simulink library "ddm"  (R2021b)
settings: Solver=VariableStepAuto  StartTime=0.0  StopTime=10.0  RelTol=1e-3
undefined symbols (not defined in the file or in its folder): ENUM_ADASACCSTA_ERROR, ENUM_ADASACCSTA_OFF, ENUM_ADASACCSTA_STANDBY, ENUM_ADASISASTA_OFF, ENUM_ALLOWMOV_ALLOWREADY, ENUM_APS, ENUM_BRKSTA_ERROR, ENUM_BRKSTA_OFF, ENUM_BRKSTA_ON, ENUM_BRKSW_INVALID, ENUM_BRKSW_OFF, ENUM_BRKSW_ON, ENUM_CHGPREACTERRSTA_OBCPRE, ENUM_DCDCFAULTSTA_ANYFAULTLV1, ENUM_DCDCFAULTSTA_ANYFAULTLV2, ENUM_DRIVETRAIN_AWD, ENUM_DRIVETRAIN_FWD, ENUM_DRIVETRAIN_RWD, ENUM_DRSEATSTA_INVALID, ENUM_EDUDRTSTA_NORMAL, ENUM_EPBSTA_APPLIED, ENUM_EPBSTA_RELEASED, ENUM_HVBATTREADYPRE_READY, ENUM_MCUWARN_LV0, ENUM_MCUWARN_LV1, ENUM_MCUWARN_LV2, ENUM_MCUWARN_LV3, ENUM_MCUWARN_NOERROR, ENUM_OBCFAULTSTA_ANYFAULT, ENUM_PAS_R2F2, ENUM_PDFAULT_BATTPDFAIL, ENUM_PDFAULT_DCDCDISABLE, ENUM_PDFAULT_MCUDISABLE, ENUM_PDFAULT_MCUDISCHRG, ENUM_POWERSTA_OFF, ENUM_POWERSTA_ON, ENUM_POWERSTA_READY, ENUM_POWERSTA_STANDBY, ENUM_PRESSINDI_LOW, ENUM_PUFAULT_BATTUPFAIL, ENUM_PUFAULT_DCDCENABLEFAIL, ENUM_PUFAULT_PRECHRGCHKFAIL, ENUM_PUFAULT_SAFETYCHKFAIL, ENUM_PUSTATE_COMPLETED, ENUM_PWRSTASW_OFF, ENUM_PWRSTASW_OFFA, ENUM_PWRSTASW_OFFCHVCHRG, ENUM_PWRSTASW_OFFCLVCHRG, ENUM_PWRSTASW_ON, ENUM_PWRSTASW_ONHVCHRG, ENUM_PWRSTASW_READY, ENUM_PWRSTASW_STANDBY, ENUM_RANGESTA_12IN, ENUM_SHIFTCOMMAND_D, ENUM_SHIFTCOMMAND_N, ENUM_SHIFTCOMMAND_P, ENUM_SHIFTCOMMAND_R, ENUM_VEHMALFUNLV_2ND, ENUM_VEHMALFUNLV_3RD, ENUM_VEHMALFUNLV_4TH ... (+835)
libraries: hcu_lib x750, $bdroot x12, simulink x5
(part 19 of 28)

== system ddm/DDM/DDM/PMM/LV/LV power supply voltage too high ==
  note: Diagnostics and Fault Handling
  note: Release Condition After Decision
  note: Test Pass Criteria
  note: Fail Safe After Decision
  note: Test Detection Criteria
  note: Fail Safe During Detection
  note: Release Condition During Detection
  task_time_s : Inport
  VPMM_PowerSta_enum : Inport  Port=2
  VPMM_PwrStaSW_enum : Inport  Port=3
  VINP_LVBattDet12V_V : Inport  Port=4
  VINP_CANMsgValidBMS2_flg : Inport  Port=5
  DTC_clear_request : Inport  Port=6
  Constant1 : Constant  Value=TRUE
  Constant10 : Constant  Value=ENUM_POWERSTA_OFF
  Constant11 : Constant  Value=KDDM_LVSupHiPassSW_flg
  Constant12 : Constant  Value=ENUM_PWRSTASW_READY
  Constant13 : Constant  Value=ENUM_PWRSTASW_ON
  Constant14 : Constant  Value=ENUM_PWRSTASW_OFFCLVCHRG
  Constant15 : Constant  Value=KDDM_LVSupHiCFSSW_flg
  Constant16 : Constant  Value=TRUE
  Constant17 : Constant  Value=ENUM_PWRSTASW_OFFCHVCHRG
  Constant18 : Constant  Value=KDDM_LVSupHiPassTO_s
  Constant19 : Constant  Value=KDDM_LVSupHiPassTO_s
  Constant2 : Constant  Value=ENUM_PWRSTASW_ON
  Constant20 : Constant  Value=KDDM_LVSupHiDFSSW_flg
  Constant{4,21,25,27} (4 alike) : Constant  Value=FALSE
  Constant22 : Constant  Value=ENUM_PWRSTASW_OFFCLVCHRG
  Constant23 : Constant  Value=ENUM_PWRSTASW_ONHVCHRG
  Constant24 : Constant  Value=TRUE
  Constant26 : Constant  Value=ENUM_PWRSTASW_OFFA
  Constant3 : Constant  Value=ENUM_PWRSTASW_ONHVCHRG
  Constant40 : Constant  Value=KDDM_LVSupHiDTC_cnt
  Constant41 : Constant  Value=KDDM_LVSupHiDetTO_s
  Constant46 : Constant  Value=KDDM_LVSupHiDetSW_flg
  Constant48 : Constant  Value=KDDM_LVSupHiDTC_cnt
  Constant5 : Constant  Value=ENUM_PWRSTASW_READY
  Constant6 : Constant  Value=KDDM_LVSupHiThd_mv
  Constant7 : Constant  Value=ENUM_PWRSTASW_OFFCHVCHRG
  Constant8 : Constant  Value=ENUM_PWRSTASW_OFFA
  Constant9 : Constant  Value=KDDM_LVSupHiThd_mv
  DTC_Couter : hcu_lib/Basic_Blocks/DTC_Couter
  DTC_Info : hcu_lib/Basic_Blocks/DTC_Info
  Data Type Conversion1 : DataTypeConversion  OutDataTypeStr=uint8
  Equal{,1..2,4,6,8..15} (13 alike) : RelationalOperator  Operator===  OutDataTypeStr=boolean  RndMeth=Simplest
  Equal3 : RelationalOperator  OutDataTypeStr=boolean  RndMeth=Simplest
  Equal5 : RelationalOperator  OutDataTypeStr=boolean  RndMeth=Simplest
  Equal7 : RelationalOperator  OutDataTypeStr=boolean  RndMeth=Simplest
  Gain1 : Gain  Gain=KXX2XX
  Gain2 : Gain  Gain=KXX2XX
  Goto6 : Goto  Commented=on  GotoTag=VDDM_EDriveSysErrVCUErr_flg
  Logical Operator{1..2,12,15,18} (5 alike) : Logic  AllPortsSameDT=off  OutDataTypeStr=boolean
  Logical Operator19 : Logic  Inputs=3  AllPortsSameDT=off  OutDataTypeStr=boolean
  Logical Operator3 : Logic  Operator=OR  Inputs=3  AllPortsSameDT=off  OutDataTypeStr=boolean
  Logical Operator4 : Logic  Operator=NOT  AllPortsSameDT=off  OutDataTypeStr=boolean
  Logical Operator5 : Logic  Operator=OR  AllPortsSameDT=off  OutDataTypeStr=boolean
  Logical Operator6 : Logic  Operator=NOT  AllPortsSameDT=off  OutDataTypeStr=boolean
  Logical Operator7 : Logic  Operator=OR  AllPortsSameDT=off  OutDataTypeStr=boolean
  Logical Operator8 : Logic  Operator=OR  AllPortsSameDT=off  OutDataTypeStr=boolean
  OR : Logic  Operator=OR  Inputs=6  AllPortsSameDT=off  OutDataTypeStr=boolean
  OR1 : Logic  Operator=OR  Inputs=6  AllPortsSameDT=off  OutDataTypeStr=boolean
  Relay : Relay  OnSwitchValue=ONE_INT  OffSwitchValue=ZERO_INT
  SR_Latch1 : Subsystem  mask(SR_Latch){}
      mask help: SR latch function.
  SR_Latch3 : hcu_lib/Basic_Blocks/SR_Latch
  SR_Latch4 : hcu_lib/Basic_Blocks/SR_Latch
  Switch{,2..4,6} (5 alike) : Switch  Criteria=u2 ~= 0
  Test Detection Criteria : hcu_lib/Basic_Blocks/Test Detection Criteria
  Timer1 : hcu_lib/Basic_Blocks/Timer
  VDDM_LVSupHiDTC_raw32 : Outport
  wires:
  DTC_Couter/2 -> Data Type Conversion1/1
  [DTC_clear_request] -> Logical Operator7/2
  Logical Operator5/1 -> SR_Latch4/2
  Logical Operator18/1 -> [VDDM_LVSupHiCFS_flg]  "VDDM_LVSupHiCFS_flg"
  Logical Operator7/1 -> SR_Latch3/2
  [DTC_clear_request] -> Logical Operator4/1
  [DTC_clear_request] -> Logical Operator5/2
  Logical Operator3/1 -> Logical Operator15/1
  Constant48/1 -> DTC_Couter/3
  [DTC_clear_request] -> Logical Operator3/3
  Logical Operator4/1 -> Logical Operator19/3
  [VDDM_LVSupHiCFS_flg] -> Logical Operator7/1
  [VDDM_LVSupHiDTC_cnt] -> Relay/1
  Constant15/1 -> Logical Operator18/2
  DTC_Couter/1 -> SR_Latch4/1
  Logical Operator12/1 -> [VDDM_LVSupHiDFS_flg]  "VDDM_LVSupHiDFS_flg"
  Logical Operator15/1 -> DTC_Couter/2
  [VDDM_LVSupHiCFSRls_flg] -> Logical Operator3/2
  Data Type Conversion1/1 -> [VDDM_LVSupHiDTC_cnt]  "VDDM_LVSupHiDTC_cnt"
  Constant46/1 -> Logical Operator19/2
  Relay/1 -> SR_Latch3/1
  SR_Latch4/1 -> Logical Operator18/1
  [VDDM_LVSupHiPass_flg] -> Logical Operator3/1
  Logical Operator19/1 -> DTC_Couter/1
  [VDDM_LVSupHiDet_flg] -> Logical Operator19/1
  Constant20/1 -> Logical Operator12/1
  [VDDM_LVSupHiCFSRls_flg] -> Logical Operator5/1
  SR_Latch3/1 -> Logical Operator12/2
  Constant11/1 -> Logical Operator15/2
  [VDDM_xxx_flg] -> SR_Latch1/2(reset)
  Constant27/1 -> Switch6/1
  Switch3/1 -> Switch6/3, [VDDM_xxx_flg]
  Switch6/1 -> Test Detection Criteria/1
  [DTC_clear_request] -> Switch6/2
  [DTC_clear_request] -> DTC_Info/4
  Constant7/1 -> Equal10/1
  Equal14/1 -> OR1/4
  [VPMM_PwrStaSW_enum] -> Equal2/1, Equal6/2
  Constant13/1 -> Equal6/1
  Logical Operator1/1 -> Switch4/2
  Equal15/1 -> OR1/3
  Constant5/1 -> Equal15/1
  [VPMM_PwrStaSW_enum] -> Equal14/1, Equal15/2
  OR1/1 -> Logical Operator1/1
  Equal6/1 -> OR1/1
  [VINP_CANMsgValidBMS2_flg] -> Logical Operator1/2
  Equal2/1 -> OR1/2
  Constant26/1 -> Equal14/2
  Constant23/1 -> Equal2/2
  Equal11/1 -> OR1/6
  [VPMM_PwrStaSW_enum] -> Equal11/1, Equal10/2
  Constant14/1 -> Equal11/2
  Equal10/1 -> OR1/5
  Constant17/1 -> Equal12/1
  Equal8/1 -> OR/4
  [VPMM_PwrStaSW_enum] -> Equal/1, Equal1/2
  Constant2/1 -> Equal1/1
  Logical Operator2/1 -> Switch3/2
  Equal9/1 -> OR/3
  Constant12/1 -> Equal9/1
  [VPMM_PwrStaSW_enum] -> Equal8/1, Equal9/2
  OR/1 -> Logical Operator2/1
  Equal1/1 -> OR/1
  [VINP_CANMsgValidBMS2_flg] -> Logical Operator2/2
  Equal/1 -> OR/2
  Constant8/1 -> Equal8/2
  Constant3/1 -> Equal/2
  Equal13/1 -> OR/6
  [VPMM_PwrStaSW_enum] -> Equal13/1, Equal12/2
  Constant22/1 -> Equal13/2
  Equal12/1 -> OR/5
  Constant41/1 -> Test Detection Criteria/4
  [VDDM_LVSupHiDet_flg] -> DTC_Info/1
  [VDDM_LVSupHiCFS_flg] -> DTC_Info/3
  [VDDM_LVSupHiPass_flg] -> DTC_Info/2
  DTC_Info/1 -> VDDM_LVSupHiDTC_raw32/1  "VDDM_LVSupHiDTC_raw32"
  VPMM_PwrStaSW_enum/1 -> [VPMM_PwrStaSW_enum]
  VPMM_PowerSta_enum/1 -> [VPMM_PowerSta_enum]
  [task_time_s] -> Timer1/3
  Constant6/1 -> Equal5/2
  Constant19/1 -> Equal3/2
  Logical Operator6/1 -> Timer1/1
  [VPMM_PowerSta_enum] -> Equal4/1
  Equal5/1 -> Switch3/1
  Constant25/1 -> Switch2/3
  Constant16/1 -> Switch4/3
  [DTC_clear_request] -> Logical Operator8/2
  Equal7/1 -> Switch4/1
  Gain1/1 -> Equal5/1
  Switch2/1 -> [VDDM_LVSupHiCFSRls_flg]  "VDDM_LVSupHiCFSRls_flg"
  [VINP_LVBattDet12V_V] -> Gain1/1
  Constant18/1 -> Timer1/4
  [VINP_LVBattDet12V_V] -> Gain2/1
  Gain2/1 -> Equal7/1
  Constant9/1 -> Equal7/2
  Constant40/1 -> Test Detection Criteria/3
  Constant1/1 -> Switch/1
  Switch4/1 -> Timer1/2, Logical Operator6/1
  Logical Operator8/1 -> Switch2/2
  Constant24/1 -> Switch2/1
  Constant10/1 -> Equal4/2
  Constant21/1 -> Switch/3
  [VDDM_LVSupHiCFS_flg] -> Switch/2
  Equal4/1 -> Logical Operator8/1
  Switch/1 -> Goto6/1
  Timer1/1 -> Equal3/1
  [task_time_s] -> Test Detection Criteria/2
  Test Detection Criteria/1 -> [VDDM_LVSupHiDet_flg]  "VDDM_LVSupHiDet_flg"
  Constant4/1 -> Switch3/3
  SR_Latch1/1(latched) -> [VDDM_LVSupHiPass_flg]  "VDDM_LVSupHiPass_flg"
  Equal3/1 -> SR_Latch1/1(set)
  VINP_CANMsgValidBMS2_flg/1 -> [VINP_CANMsgValidBMS2_flg]
  DTC_clear_request/1 -> [DTC_clear_request]
  VINP_LVBattDet12V_V/1 -> [VINP_LVBattDet12V_V]
  task_time_s/1 -> [task_time_s]

== system ddm/DDM/DDM/PMM/LV/LV power supply voltage too low ==
  note: Diagnostics and Fault Handling
  note: Release Condition After Decision
  note: Release Condition During Detection
  note: Fail Safe During Detection
  note: Fail Safe After Decision
  note: Test Pass Criteria
  note: Test Detection Criteria
  task_time_s : Inport
  VPMM_PowerSta_enum : Inport  Port=2
  VPMM_PwrStaSW_enum : Inport  Port=3
  VINP_LVBattDet12V_V : Inport  Port=4
  VINP_CANMsgValidBMS2_flg : Inport  Port=5
  DTC_clear_request : Inport  Port=6
  Constant1 : Constant  Value=TRUE
  Constant10 : Constant  Value=ENUM_POWERSTA_OFF
  Constant11 : Constant  Value=KDDM_LVSupLoPassSW_flg
  Constant12 : Constant  Value=ENUM_PWRSTASW_READY
  Constant13 : Constant  Value=ENUM_PWRSTASW_ON
  Constant14 : Constant  Value=ENUM_PWRSTASW_OFFCLVCHRG
  Constant15 : Constant  Value=KDDM_LVSupLoCFSSW_flg
  Constant16 : Constant  Value=TRUE
  Constant17 : Constant  Value=ENUM_PWRSTASW_OFFCHVCHRG
  Constant18 : Constant  Value=KDDM_LVSupLoPassTO_s
  Constant19 : Constant  Value=KDDM_LVSupLoPassTO_s
  Constant2 : Constant  Value=ENUM_PWRSTASW_ON
  Constant20 : Constant  Value=KDDM_LVSupLoDFSSW_flg
  Constant{4,21,25,27} (4 alike) : Constant  Value=FALSE
  Constant22 : Constant  Value=ENUM_PWRSTASW_OFFCLVCHRG
  Constant23 : Constant  Value=ENUM_PWRSTASW_ONHVCHRG
  Constant24 : Constant  Value=TRUE
  Constant26 : Constant  Value=ENUM_PWRSTASW_OFFA
  Constant3 : Constant  Value=ENUM_PWRSTASW_ONHVCHRG
  Constant40 : Constant  Value=KDDM_LVSupLoDTC_cnt
  Constant41 : Constant  Value=KDDM_LVSupLoDetTO_s
  Constant46 : Constant  Value=KDDM_LVSupLoDetSW_flg
  Constant48 : Constant  Value=KDDM_LVSupLoDTC_cnt
  Constant5 : Constant  Value=ENUM_PWRSTASW_READY
  Constant6 : Constant  Value=KDDM_LVSupLoThd_mv
  Constant7 : Constant  Value=ENUM_PWRSTASW_OFFCHVCHRG
  Constant8 : Constant  Value=ENUM_PWRSTASW_OFFA
  Constant9 : Constant  Value=KDDM_LVSupLoThd_mv
  DTC_Couter : hcu_lib/Basic_Blocks/DTC_Couter
  DTC_Info : hcu_lib/Basic_Blocks/DTC_Info
  Data Type Conversion1 : DataTypeConversion  OutDataTypeStr=uint8
  Equal{,1..2,4,6,8..15} (13 alike) : RelationalOperator  Operator===  OutDataTypeStr=boolean  RndMeth=Simplest
  Equal3 : RelationalOperator  OutDataTypeStr=boolean  RndMeth=Simplest
  Equal5 : RelationalOperator  Operator=<=  OutDataTypeStr=boolean  RndMeth=Simplest
  Equal7 : RelationalOperator  Operator=<=  OutDataTypeStr=boolean  RndMeth=Simplest
  Gain1 : Gain  Gain=1000
  Gain2 : Gain  Gain=1000
  Goto6 : Goto  Commented=on  GotoTag=VDDM_EDriveSysErrVCUErr_flg
  Logical Operator{1..2,12,15,18} (5 alike) : Logic  AllPortsSameDT=off  OutDataTypeStr=boolean
  Logical Operator19 : Logic  Inputs=3  AllPortsSameDT=off  OutDataTypeStr=boolean
  Logical Operator3 : Logic  Operator=OR  Inputs=3  AllPortsSameDT=off  OutDataTypeStr=boolean
  Logical Operator4 : Logic  Operator=NOT  AllPortsSameDT=off  OutDataTypeStr=boolean
  Logical Operator5 : Logic  Operator=OR  AllPortsSameDT=off  OutDataTypeStr=boolean
  Logical Operator6 : Logic  Operator=NOT  AllPortsSameDT=off  OutDataTypeStr=boolean
  Logical Operator7 : Logic  Operator=OR  AllPortsSameDT=off  OutDataTypeStr=boolean
  Logical Operator8 : Logic  Operator=OR  AllPortsSameDT=off  OutDataTypeStr=boolean
  OR : Logic  Operator=OR  Inputs=6  AllPortsSameDT=off  OutDataTypeStr=boolean
  OR1 : Logic  Operator=OR  Inputs=6  AllPortsSameDT=off  OutDataTypeStr=boolean
  Relay : Relay  OnSwitchValue=ONE_INT  OffSwitchValue=ZERO_INT
  SR_Latch1 : Subsystem  mask(SR_Latch){}
      mask help: SR latch function.
  SR_Latch3 : hcu_lib/Basic_Blocks/SR_Latch
  SR_Latch4 : hcu_lib/Basic_Blocks/SR_Latch
  Switch{,2..4,6} (5 alike) : Switch  Criteria=u2 ~= 0
  Test Detection Criteria : hcu_lib/Basic_Blocks/Test Detection Criteria
  Timer1 : hcu_lib/Basic_Blocks/Timer
  VDDM_LVSupLoDTC_raw32 : Outport
  wires:
  Constant46/1 -> Logical Operator19/2
  Logical Operator12/1 -> [VDDM_LVSupLoDFS_flg]  "VDDM_LVSupLoDFS_flg"
  Logical Operator5/1 -> SR_Latch4/2
  [VDDM_LVSupLoPass_flg] -> Logical Operator3/1
  Constant11/1 -> Logical Operator15/2
  Data Type Conversion1/1 -> [VDDM_LVSupLoDTC_cnt]  "VDDM_LVSupLoDTC_cnt"
  [DTC_clear_request] -> Logical Operator4/1
  SR_Latch3/1 -> Logical Operator12/2
  Logical Operator4/1 -> Logical Operator19/3
  Constant20/1 -> Logical Operator12/1
  Logical Operator19/1 -> DTC_Couter/1
  Logical Operator18/1 -> [VDDM_LVSupLoCFS_flg]  "VDDM_LVSupLoCFS_flg"
  [DTC_clear_request] -> Logical Operator5/2
  DTC_Couter/2 -> Data Type Conversion1/1
  Logical Operator3/1 -> Logical Operator15/1
  Constant48/1 -> DTC_Couter/3
  [VDDM_LVSupLoDet_flg] -> Logical Operator19/1
  [VDDM_LVSupLoDTC_cnt] -> Relay/1
  [DTC_clear_request] -> Logical Operator3/3
  Logical Operator7/1 -> SR_Latch3/2
  [VDDM_LVSupLoCFS_flg] -> Logical Operator7/1
  Logical Operator15/1 -> DTC_Couter/2
  Relay/1 -> SR_Latch3/1
  DTC_Couter/1 -> SR_Latch4/1
  SR_Latch4/1 -> Logical Operator18/1
  Constant15/1 -> Logical Operator18/2
  [DTC_clear_request] -> Logical Operator7/2
  [VDDM_LVSupLoCFSRls_flg] -> Logical Operator3/2
  [VDDM_LVSupLoCFSRls_flg] -> Logical Operator5/1
  [VDDM_xxx_flg] -> SR_Latch1/2(reset)
  Constant27/1 -> Switch6/1
  Switch3/1 -> Switch6/3, [VDDM_xxx_flg]
  Switch6/1 -> Test Detection Criteria/1
  [DTC_clear_request] -> Switch6/2
  [DTC_clear_request] -> DTC_Info/4
  Constant7/1 -> Equal10/1
  Equal14/1 -> OR1/4
  [VPMM_PwrStaSW_enum] -> Equal2/1, Equal6/2
  Constant13/1 -> Equal6/1
  Logical Operator1/1 -> Switch4/2
  Equal15/1 -> OR1/3
  Constant5/1 -> Equal15/1
  [VPMM_PwrStaSW_enum] -> Equal14/1, Equal15/2
  OR1/1 -> Logical Operator1/1
  Equal6/1 -> OR1/1
  [VINP_CANMsgValidBMS2_flg] -> Logical Operator1/2
  Equal2/1 -> OR1/2
  Constant26/1 -> Equal14/2
  Constant23/1 -> Equal2/2
  Equal11/1 -> OR1/6
  [VPMM_PwrStaSW_enum] -> Equal11/1, Equal10/2
  Constant14/1 -> Equal11/2
  Equal10/1 -> OR1/5
  Equal13/1 -> OR/6
  Equal12/1 -> OR/5
  Constant22/1 -> Equal13/2
  Constant17/1 -> Equal12/1
  [VPMM_PwrStaSW_enum] -> Equal13/1, Equal12/2
  Constant41/1 -> Test Detection Criteria/4
  [VDDM_LVSupLoDet_flg] -> DTC_Info/1
  [VDDM_LVSupLoCFS_flg] -> DTC_Info/3
  [VDDM_LVSupLoPass_flg] -> DTC_Info/2
  DTC_Info/1 -> VDDM_LVSupLoDTC_raw32/1  "VDDM_LVSupLoDTC_raw32"
  [VPMM_PowerSta_enum] -> Equal4/1
  [task_time_s] -> Timer1/3
  Equal8/1 -> OR/4
  Equal9/1 -> OR/3
  Constant12/1 -> Equal9/1
  [VPMM_PwrStaSW_enum] -> Equal8/1, Equal9/2
  Constant8/1 -> Equal8/2
  Constant9/1 -> Equal7/2
  [VINP_LVBattDet12V_V] -> Gain2/1
  Gain2/1 -> Equal7/1
  Equal7/1 -> Switch4/1
  Gain1/1 -> Equal5/1
  Constant6/1 -> Equal5/2
  Equal5/1 -> Switch3/1
  [VINP_LVBattDet12V_V] -> Gain1/1
  Constant2/1 -> Equal1/1
  Equal1/1 -> OR/1
  OR/1 -> Logical Operator2/1
  Equal/1 -> OR/2
  [VINP_CANMsgValidBMS2_flg] -> Logical Operator2/2
  VINP_CANMsgValidBMS2_flg/1 -> [VINP_CANMsgValidBMS2_flg]
  DTC_clear_request/1 -> [DTC_clear_request]
  Equal4/1 -> Logical Operator8/1
  Constant10/1 -> Equal4/2
  Constant24/1 -> Switch2/1
  [DTC_clear_request] -> Logical Operator8/2
  Switch2/1 -> [VDDM_LVSupLoCFSRls_flg]  "VDDM_LVSupLoCFSRls_flg"
  Constant25/1 -> Switch2/3
  Logical Operator8/1 -> Switch2/2
  Constant21/1 -> Switch/3
  Constant1/1 -> Switch/1
  Switch/1 -> Goto6/1
  [VDDM_LVSupLoCFS_flg] -> Switch/2
  Constant16/1 -> Switch4/3
  Constant18/1 -> Timer1/4
  Timer1/1 -> Equal3/1
  Switch4/1 -> Timer1/2, Logical Operator6/1
  Constant19/1 -> Equal3/2
  Logical Operator6/1 -> Timer1/1
  Equal3/1 -> SR_Latch1/1(set)
  SR_Latch1/1(latched) -> [VDDM_LVSupLoPass_flg]  "VDDM_LVSupLoPass_flg"
  [VPMM_PwrStaSW_enum] -> Equal/1, Equal1/2
  Constant4/1 -> Switch3/3
  Constant3/1 -> Equal/2
  Constant40/1 -> Test Detection Criteria/3
  Test Detection Criteria/1 -> [VDDM_LVSupLoDet_flg]  "VDDM_LVSupLoDet_flg"
  [task_time_s] -> Test Detection Criteria/2
  Logical Operator2/1 -> Switch3/2
  VPMM_PowerSta_enum/1 -> [VPMM_PowerSta_enum]
  VPMM_PwrStaSW_enum/1 -> [VPMM_PwrStaSW_enum]
  VINP_LVBattDet12V_V/1 -> [VINP_LVBattDet12V_V]
  task_time_s/1 -> [task_time_s]

== system ddm/DDM/DDM/PMM/SW failure/Driver seat switch failure ==
  note: Diagnostics and Fault Handling
  note: Release Condition During Detection
  note: Release Condition After Decision
  note: Fail Safe After Decision
  note: Fail Safe During Detection
  note: Test Detection Criteria
  note: Test Pass Criteria
  task_time_s : Inport
  VPMM_PowerSta_enum : Inport  Port=2
  VPMM_PwrStaSW_enum : Inport  Port=3
  VINP_DrStSW : Inport  Port=4
  DTC_clear_request : Inport  Port=5
  Constant15 : Constant  Value=KDDM_DrStSWDetTO_s
  Constant16 : Constant  Value=KDDM_DrStSWDTC_cnt
  Constant17 : Constant  Value=KDDM_DrStSWPassTO_s
  Constant18 : Constant  Value=FALSE
  Constant19 : Constant  Value=ENUM_PWRSTASW_OFF
  Constant20 : Constant  Value=KDDM_DrStSWPassTO_s
  Constant21 : Constant  Value=ZERO_INT
  Constant22 : Constant  Value=ENUM_PWRSTASW_OFF
  Constant23 : Constant  Value=TRUE
  Constant24 : Constant  Value=KDDM_DrStSWPassTO_s
  Constant26 : Constant  Value=ONE_INT
  Constant27 : Constant  Value=KDDM_DrStSW_s
  Constant42 : Constant  Value=ENUM_DRSEATSTA_INVALID
  Constant45 : Constant  Value=ENUM_POWERSTA_OFF
  Constant52 : Constant  Value=TRUE
  Constant53 : Constant  Value=FALSE
  Constant54 : Constant  Value=TRUE
  Constant55 : Constant  Value=FALSE
  Constant56 : Constant  Value=KDDM_DrStSWPassSW_flg
  Constant57 : Constant  Value=KDDM_DrStSWCFSSW_flg
  Constant58 : Constant  Value=KDDM_DrStSWDFSSW_flg
  Constant59 : Constant  Value=KDDM_DrStSWDetSW_flg
  Constant60 : Constant  Value=KDDM_DrStSWDTC_cnt
  Constant8 : Constant  Value=ZERO_FLOAT
  DTC_Couter1 : hcu_lib/Basic_Blocks/DTC_Couter
  DTC_Info : hcu_lib/Basic_Blocks/DTC_Info
  Data Type Conversion11 : DataTypeConversion
  Data Type Conversion12 : DataTypeConversion  OutDataTypeStr=boolean
  Data Type Conversion4 : DataTypeConversion  OutDataTypeStr=uint8
  Equal1 : RelationalOperator  Operator=~=  OutDataTypeStr=boolean  RndMeth=Simplest
  Equal2 : RelationalOperator  Operator=~=  OutDataTypeStr=boolean  RndMeth=Simplest
  Equal3 : RelationalOperator  Operator=~=  OutDataTypeStr=boolean  RndMeth=Simplest
  Equal5 : RelationalOperator  OutDataTypeStr=boolean  RndMeth=Simplest
  Equal8 : RelationalOperator  Operator===  OutDataTypeStr=boolean  RndMeth=Simplest
  Logical Operator{2,4..5,7} (4 alike) : Logic  Operator=NOT  AllPortsSameDT=off  OutDataTypeStr=boolean
  Logical Operator27 : Logic  Operator=OR  AllPortsSameDT=off  OutDataTypeStr=boolean
  Logical Operator{6,28..30} (4 alike) : Logic  AllPortsSameDT=off  OutDataTypeStr=boolean
  Logical Operator3 : Logic  Operator=OR  AllPortsSameDT=off  OutDataTypeStr=boolean
  Logical Operator31 : Logic  Inputs=3  AllPortsSameDT=off  OutDataTypeStr=boolean
  Logical Operator32 : Logic  Operator=OR  Inputs=3  AllPortsSameDT=off  OutDataTypeStr=boolean
  Logical Operator33 : Logic  Operator=OR  Inputs=3  AllPortsSameDT=off  OutDataTypeStr=boolean
  Relational Operator3 : RelationalOperator  Operator=>  OutDataTypeStr=boolean  RndMeth=Simplest
  Relational Operator4 : RelationalOperator  Operator=<=  OutDataTypeStr=boolean  RndMeth=Simplest
  Relay1 : Relay  OnSwitchValue=ONE_INT  OffSwitchValue=ZERO_INT
  SR_Latch1 : hcu_lib/Basic_Blocks/SR_Latch
  SR_Latch2 : hcu_lib/Basic_Blocks/SR_Latch
  SR_Latch3 : Subsystem  mask(SR_Latch){}
      mask help: SR latch function.
  SR_Latch5 : hcu_lib/Basic_Blocks/SR_Latch
  Subsystem : Subsystem
  Switch{5,10..11,14..16} (6 alike) : Switch  Criteria=u2 ~= 0
  Test Detection Criteria2 : hcu_lib/Basic_Blocks/Test Detection Criteria
  Timer : hcu_lib/Basic_Blocks/Test Detection Criteria/Timer
  Timer1 : hcu_lib/Basic_Blocks/Timer
  Unit Delay : UnitDelay  SampleTime=-1  HasFrameUpgradeWarning=on
  Unit Delay7 : UnitDelay  SampleTime=-1  HasFrameUpgradeWarning=on
  VDDM_DrStSWDTC_raw32 : Outport
  VDDM_DrSeatSta_enum : Outport  Port=2
  wires:
  [DTC_clear_request] -> Logical Operator32/3
  [DTC_clear_request] -> Logical Operator33/3
  [DTC_clear_request] -> Logical Operator3/2
  Constant57/1 -> Logical Operator30/2
  Logical Operator2/1 -> Logical Operator31/3
  Constant59/1 -> Logical Operator31/2
  Logical Operator3/1 -> SR_Latch5/2
  [DTC_clear_request] -> Logical Operator2/1
  Logical Operator28/1 -> [VDDM_DrStSWDFS_flg]  "VDDM_DrStSWDFS_flg"
  Logical Operator32/1 -> SR_Latch2/2
  DTC_Couter1/1 -> SR_Latch5/1
  [VDDM_DrStSWCFSRls_flg] -> Logical Operator33/2
  [VDDM_DrStSWDFSRls_flg] -> Logical Operator32/1
  SR_Latch5/1 -> Logical Operator30/1
  Logical Operator31/1 -> DTC_Couter1/1
  [VDDM_DrStSWDTC_cnt] -> Relay1/1
  Relay1/1 -> SR_Latch2/1
  SR_Latch2/1 -> Logical Operator28/2
  Constant60/1 -> DTC_Couter1/3
  [VDDM_DrStSWDet_flg] -> Logical Operator31/1
  [VDDM_DrStSWCFSRls_flg] -> Logical Operator3/1
  Logical Operator33/1 -> Logical Operator29/1
  Constant58/1 -> Logical Operator28/1
  Constant56/1 -> Logical Operator29/2
  [VDDM_DrStSWPass_flg] -> Logical Operator33/1
  Logical Operator29/1 -> DTC_Couter1/2
  DTC_Couter1/2 -> Data Type Conversion4/1
  Data Type Conversion4/1 -> [VDDM_DrStSWDTC_cnt]  "VDDM_DrStSWDTC_cnt"
  [VDDM_DrStSWCFS_flg] -> Logical Operator32/2
  Logical Operator30/1 -> [VDDM_DrStSWCFS_flg]  "VDDM_DrStSWCFS_flg"
  [DTC_clear_request] -> DTC_Info/4
  [VDDM_DrStSWDet_flg] -> DTC_Info/1
  [VDDM_DrStSWCFS_flg] -> DTC_Info/3
  [VDDM_DrStSWPass_flg] -> DTC_Info/2
  DTC_Info/1 -> VDDM_DrStSWDTC_raw32/1  "VDDM_DrStSWDTC_raw32"
  [VINP_DrStSWGPIO_flg] -> Switch11/3
  VPMM_PwrStaSW_enum/1 -> [VPMM_PwrStaSW_enum]
  VPMM_PowerSta_enum/1 -> [VPMM_PowerSta_enum]
  [VDDM_DrSeatSta_enum] -> VDDM_DrSeatSta_enum/1
  [VPMM_PowerSta_enum] -> Equal8/1
  Constant54/1 -> Switch15/1
  [DTC_clear_request] -> Logical Operator27/2
  Switch16/1 -> [VDDM_DrStSWDFSRls_flg]  "VDDM_DrStSWDFSRls_flg"
  Switch15/1 -> [VDDM_DrStSWCFSRls_flg]  "VDDM_DrStSWCFSRls_flg"
  Constant55/1 -> Switch15/3
  Constant45/1 -> Equal8/2
  Constant53/1 -> Switch16/3
  [VDDM_DrStSWPass_flg] -> Switch16/2
  Equal8/1 -> Logical Operator27/1
  Constant52/1 -> Switch16/1
  Logical Operator27/1 -> Switch15/2
  Switch11/1 -> [VDDM_DrSeatSta_enum]  "VDDM_DrSeatSta_enum"
  Constant42/1 -> Switch11/1
  [VDDM_DrStSWCFS_flg] -> Switch11/2
  task_time_s/1 -> [task_time_s]
  VINP_DrStSW/1 -> [VINP_DrStSWGPIO_flg]
  DTC_clear_request/1 -> [DTC_clear_request]
  SR_Latch1/1 -> Logical Operator5/1, Logical Operator4/1, Timer/1
  Constant17/1 -> Timer/4
  Timer/1 -> Relational Operator4/1, Unit Delay/1
  [VDDM_xxx_flg] -> SR_Latch3/2(reset)
  [DTC_clear_request] -> Switch5/2
  Switch5/1 -> Data Type Conversion12/1
  Constant18/1 -> Switch5/1
  Constant15/1 -> Data Type Conversion11/1
  Constant26/1 -> SR_Latch1/1
  Logical Operator5/1 -> Subsystem/Trigger
  Constant20/1 -> Equal5/2
  [DrStSWFault_flg] -> Switch10/1
  Switch14/1 -> [VDDM_xxx_flg], Switch5/3
  Test Detection Criteria2/1 -> [VDDM_DrStSWDet_flg]  "VDDM_DrStSWDet_flg"
  [VPMM_PwrStaSW_enum] -> Equal1/1
  Constant22/1 -> Equal1/2
  Constant21/1 -> Switch14/3
  Equal1/1 -> Switch14/2
  Data Type Conversion11/1 -> Test Detection Criteria2/4
  Equal2/1 -> [VDDM_DrStSWChange_flg]
  Logical Operator4/1 -> Timer/2
  Subsystem/1(Fault_flg) -> Logical Operator6/1
  [VDDM_DrStSWChange_flg] -> SR_Latch1/2
  Constant16/1 -> Test Detection Criteria2/3
  Relational Operator4/1 -> Logical Operator6/2
  [task_time_s] -> Test Detection Criteria2/2
  Logical Operator7/1 -> Timer1/1
  Equal3/1 -> Switch10/2
  Equal5/1 -> SR_Latch3/1(set)
  Switch10/1 -> Logical Operator7/1, Timer1/2
  SR_Latch3/1(latched) -> [VDDM_DrStSWPass_flg]  "VDDM_DrStSWPass_flg"
  Unit Delay/1 -> Subsystem/1(In1)
  Logical Operator6/1 -> [DrStSWFault_flg], Switch14/1
  Data Type Conversion12/1 -> Test Detection Criteria2/1
  Constant23/1 -> Switch10/3
  Constant19/1 -> Equal3/2
  Timer1/1 -> Equal5/1
  [task_time_s] -> Timer1/3
  [VPMM_PwrStaSW_enum] -> Equal3/1
  Constant8/1 -> Relational Operator3/2
  Unit Delay7/1 -> Equal2/1
  [VINP_DrStSWGPIO_flg] -> Relational Operator3/1
  Constant24/1 -> Timer1/4
  Relational Operator3/1 -> Equal2/2, Unit Delay7/1
  Constant27/1 -> Relational Operator4/2
  [task_time_s] -> Timer/3

== system ddm/DDM/DDM/PMM/SW failure/FL Door switch failure ==
  note: Diagnostics and Fault Handling
  note: Fail Safe During Detection
  note: Fail Safe After Decision
  note: Release Condition After Decision
  note: Release Condition During Detection
  note: Test Pass Criteria
  note: Test Detection Criteria
  task_time_s : Inport
  VPMM_PowerSta_enum : Inport  Port=2
  VPMM_PwrStaSW_enum : Inport  Port=3
  VINP_FLAJARSW : Inport  Port=4
  DTC_clear_request : Inport  Port=5
  Constant{10,18,53,55} (4 alike) : Constant  Value=FALSE
  Constant11 : Constant  Value=KDDM_FLDoorSWPassTO_s
  Constant15 : Constant  Value=KDDM_FLDoorSWPassTO_s
  Constant16 : Constant  Value=KDDM_FLDoorSWDetTO_s
  Constant17 : Constant  Value=KDDM_FLDoorSW_s
  Constant19 : Constant  Value=ENUM_PWRSTASW_OFF
  Constant21 : Constant  Value=ZERO_INT
  Constant22 : Constant  Value=ENUM_PWRSTASW_OFF
  Constant{23,42,52,54} (4 alike) : Constant  Value=TRUE
  Constant24 : Constant  Value=KDDM_FLDoorSWPassTO_s
  Constant25 : Constant  Value=KDDM_FLDoorSWDTC_cnt
  Constant26 : Constant  Value=ONE_INT
  Constant32 : Constant  Value=ZERO_FLOAT
  Constant45 : Constant  Value=ENUM_POWERSTA_OFF
  Constant56 : Constant  Value=KDDM_FLDoorSWPassSW_flg
  Constant57 : Constant  Value=KDDM_FLDoorSWCFSSW_flg
  Constant58 : Constant  Value=KDDM_FLDoorSWDFSSW_flg
  Constant59 : Constant  Value=KDDM_FLDoorSWDetSW_flg
  Constant60 : Constant  Value=KDDM_FLDoorSWDTC_cnt
  DTC_Couter1 : hcu_lib/Basic_Blocks/DTC_Couter
  DTC_Info : hcu_lib/Basic_Blocks/DTC_Info
  Data Type Conversion12 : DataTypeConversion  OutDataTypeStr=boolean
  Data Type Conversion14 : DataTypeConversion  OutDataTypeStr=boolean
  Data Type Conversion4 : DataTypeConversion  OutDataTypeStr=uint8
  Data Type Conversion7 : DataTypeConversion
  Equal1 : RelationalOperator  Operator=~=  OutDataTypeStr=boolean  RndMeth=Simplest
  Equal3 : RelationalOperator  Operator=~=  OutDataTypeStr=boolean  RndMeth=Simplest
  Equal4 : RelationalOperator  Operator=~=  OutDataTypeStr=boolean  RndMeth=Simplest
  Equal5 : RelationalOperator  OutDataTypeStr=boolean  RndMeth=Simplest
  Equal8 : RelationalOperator  Operator===  OutDataTypeStr=boolean  RndMeth=Simplest
  Logical Operator{2,4..5,7} (4 alike) : Logic  Operator=NOT  AllPortsSameDT=off  OutDataTypeStr=boolean
  Logical Operator27 : Logic  Operator=OR  AllPortsSameDT=off  OutDataTypeStr=boolean
  Logical Operator{6,28..30} (4 alike) : Logic  AllPortsSameDT=off  OutDataTypeStr=boolean
  Logical Operator3 : Logic  Operator=OR  AllPortsSameDT=off  OutDataTypeStr=boolean
  Logical Operator31 : Logic  Inputs=3  AllPortsSameDT=off  OutDataTypeStr=boolean
  Logical Operator32 : Logic  Operator=OR  Inputs=3  AllPortsSameDT=off  OutDataTypeStr=boolean
  Logical Operator33 : Logic  Operator=OR  Inputs=3  AllPortsSameDT=off  OutDataTypeStr=boolean
  Relational Operator4 : RelationalOperator  Operator=<=  OutDataTypeStr=boolean  RndMeth=Simplest
  Relational Operator5 : RelationalOperator  Operator=>  OutDataTypeStr=boolean  RndMeth=Simplest
  Relay1 : Relay  OnSwitchValue=ONE_INT  OffSwitchValue=ZERO_INT
  SR_Latch1 : hcu_lib/Basic_Blocks/SR_Latch
  SR_Latch2 : hcu_lib/Basic_Blocks/SR_Latch
  SR_Latch3 : $bdroot/DDM/DDM/PMM/SW failure/Driver seat switch failure/SR_Latch3
  SR_Latch5 : hcu_lib/Basic_Blocks/SR_Latch
  Subsystem : $bdroot/DDM/DDM/PMM/SW failure/Driver seat switch failure/Subsystem  SystemSampleTime=-1  VariantActivationTime=update diagram  Latency=0  AutoFrameSizeCalculation=off
      link override Constant15: Value=KDDM_FLDoorSW_s
  Switch{5,10..11,14..16} (6 alike) : Switch  Criteria=u2 ~= 0
  Test Detection Criteria2 : hcu_lib/Basic_Blocks/Test Detection Criteria
  Timer : hcu_lib/Basic_Blocks/Test Detection Criteria/Timer
  Timer1 : hcu_lib/Basic_Blocks/Timer
  Unit Delay : UnitDelay  SampleTime=-1  HasFrameUpgradeWarning=on
  Unit Delay9 : UnitDelay  SampleTime=-1  HasFrameUpgradeWarning=on
  VDDM_FLDoorSWDTC_raw32 : Outport
  VDDM_VCUFLDoorSta_flg : Outport  Port=2
  wires:
  [DTC_clear_request] -> Logical Operator3/2
  Logical Operator2/1 -> Logical Operator31/3
  [DTC_clear_request] -> Logical Operator32/3
  [DTC_clear_request] -> Logical Operator33/3
  Logical Operator29/1 -> DTC_Couter1/2
  [DTC_clear_request] -> Logical Operator2/1
  [VDDM_FLDoorSWDet_flg] -> Logical Operator31/1
  Logical Operator31/1 -> DTC_Couter1/1
  [VDDM_FLDoorSWDTC_cnt] -> Relay1/1
  Logical Operator33/1 -> Logical Operator29/1
  DTC_Couter1/1 -> SR_Latch5/1
  SR_Latch5/1 -> Logical Operator30/1
  SR_Latch2/1 -> Logical Operator28/2
  Data Type Conversion4/1 -> [VDDM_FLDoorSWDTC_cnt]  "VDDM_FLDoorSWDTC_cnt"
  DTC_Couter1/2 -> Data Type Conversion4/1
  Relay1/1 -> SR_Latch2/1
  [VDDM_FLDoorSWCFSRls_flg] -> Logical Operator3/1
  [VDDM_FLDoorSWCFS_flg] -> Logical Operator32/2
  Logical Operator28/1 -> [VDDM_FLDoorSWDFS_flg]  "VDDM_FLDoorSWDFS_flg"
  [VDDM_FLDoorSWPass_flg] -> Logical Operator33/1
  Constant60/1 -> DTC_Couter1/3
  [VDDM_FLDoorSWDFSRls_flg] -> Logical Operator32/1
  Constant56/1 -> Logical Operator29/2
  Constant58/1 -> Logical Operator28/1
  Logical Operator32/1 -> SR_Latch2/2
  Constant59/1 -> Logical Operator31/2
  [VDDM_FLDoorSWCFSRls_flg] -> Logical Operator33/2
  Logical Operator3/1 -> SR_Latch5/2
  Constant57/1 -> Logical Operator30/2
  Logical Operator30/1 -> [VDDM_FLDoorSWCFS_flg]  "VDDM_FLDoorSWCFS_flg"
  [DTC_clear_request] -> DTC_Info/4
  [VDDM_FLDoorSWDet_flg] -> DTC_Info/1
  [VDDM_FLDoorSWCFS_flg] -> DTC_Info/3
  [VDDM_FLDoorSWPass_flg] -> DTC_Info/2
  DTC_Info/1 -> VDDM_FLDoorSWDTC_raw32/1  "VDDM_FLDoorSWDTC_raw32"
  Constant10/1 -> Switch11/3
  VPMM_PowerSta_enum/1 -> [VPMM_PowerSta_enum]
  VPMM_PwrStaSW_enum/1 -> [VPMM_PwrStaSW_enum]
  DTC_clear_request/1 -> [DTC_clear_request]
  VINP_FLAJARSW/1 -> [VINP_FL_AJAR_SW]
  task_time_s/1 -> [task_time_s]
  [VDDM_FLDoorSWCFS_flg] -> Switch11/2
  Constant42/1 -> Switch11/1
  Switch11/1 -> [VDDM_VCUFLDoorSta_flg]  "VDDM_VCUFLDoorSta_flg"
  Logical Operator27/1 -> Switch15/2
  Constant52/1 -> Switch16/1
  Equal8/1 -> Logical Operator27/1
  [VDDM_FLDoorSWPass_flg] -> Switch16/2
  Constant53/1 -> Switch16/3
  Constant45/1 -> Equal8/2
  Constant55/1 -> Switch15/3
  Switch15/1 -> [VDDM_FLDoorSWCFSRls_flg]  "VDDM_FLDoorSWCFSRls_flg"
  Switch16/1 -> [VDDM_FLDoorSWDFSRls_flg]  "VDDM_FLDoorSWDFSRls_flg"
  [DTC_clear_request] -> Logical Operator27/2
  Constant54/1 -> Switch15/1
  [VPMM_PowerSta_enum] -> Equal8/1
  [VDDM_VCUFLDoorSta_flg] -> VDDM_VCUFLDoorSta_flg/1
  Switch14/1 -> [VDDM_xxx_flg], Switch5/3
  Constant26/1 -> SR_Latch1/1
  Switch5/1 -> Data Type Conversion12/1
  Constant16/1 -> Data Type Conversion7/1
  Constant18/1 -> Switch5/1
  [VDDM_xxx_flg] -> SR_Latch3/2
  SR_Latch1/1 -> Logical Operator5/1, Logical Operator4/1, Timer/1
  Constant17/1 -> Relational Operator4/2
  Constant11/1 -> Timer/4
  [DTC_clear_request] -> Switch5/2
  Timer1/1 -> Equal5/1
  Constant19/1 -> Equal3/2
  Data Type Conversion12/1 -> Test Detection Criteria2/1
  Logical Operator6/1 -> [FLDoorSWFault_flg], Switch14/1
  Unit Delay/1 -> Subsystem/1
  Timer/1 -> Relational Operator4/1, Unit Delay/1
  Logical Operator5/1 -> Subsystem/Trigger
  Switch10/1 -> Logical Operator7/1, Timer1/2
  Equal5/1 -> SR_Latch3/1
  Equal3/1 -> Switch10/2
  Constant15/1 -> Timer1/4
  Relational Operator4/1 -> Logical Operator6/2
  Constant24/1 -> Equal5/2
  Logical Operator7/1 -> Timer1/1
  [VPMM_PwrStaSW_enum] -> Equal3/1
  Subsystem/1 -> Logical Operator6/1
  [task_time_s] -> Timer1/3
  [FLDoorSWFault_flg] -> Switch10/1
  Logical Operator4/1 -> Timer/2
  Equal1/1 -> Switch14/2
  Data Type Conversion7/1 -> Test Detection Criteria2/4
  Constant23/1 -> Switch10/3
  Constant25/1 -> Test Detection Criteria2/3
  [task_time_s] -> Test Detection Criteria2/2
  [VDDM_FLDoorSWChange_flg] -> SR_Latch1/2
  Constant21/1 -> Switch14/3
  [VPMM_PwrStaSW_enum] -> Equal1/1
  [task_time_s] -> Timer/3
  Constant22/1 -> Equal1/2
  Data Type Conversion14/1 -> Equal4/1
  Equal4/1 -> [VDDM_FLDoorSWChange_flg]
  Constant32/1 -> Relational Operator5/2
  Relational Operator5/1 -> Unit Delay9/1, Equal4/2
  Unit Delay9/1 -> Data Type Conversion14/1
  [VINP_FL_AJAR_SW] -> Relational Operator5/1
  Test Detection Criteria2/1 -> [VDDM_FLDoorSWDet_flg]  "VDDM_FLDoorSWDet_flg"
  SR_Latch3/1 -> [VDDM_FLDoorSWPass_flg]  "VDDM_FLDoorSWPass_flg"

== system ddm/DDM/DDM/PMM/SW failure/FR Door switch failure ==
  note: Diagnostics and Fault Handling
  note: Release Condition During Detection
  note: Release Condition After Decision
  note: Fail Safe After Decision
  note: Fail Safe During Detection
  note: Test Pass Criteria
  note: Test Detection Criteria
  task_time_s : Inport
  VPMM_PowerSta_enum : Inport  Port=2
  VPMM_PwrStaSW_enum : Inport  Port=3
  VINP_FRAJARSW : Inport  Port=4
  DTC_clear_request : Inport  Port=5
  Constant{10,18,53,55} (4 alike) : Constant  Value=FALSE
  Constant11 : Constant  Value=KDDM_FRDoorSWPassTO_s
  Constant15 : Constant  Value=KDDM_FRDoorSWPassTO_s
  Constant16 : Constant  Value=KDDM_FRDoorSWDetTO_s
  Constant17 : Constant  Value=KDDM_FRDoorSW_s
  Constant19 : Constant  Value=ENUM_PWRSTASW_OFF
  Constant21 : Constant  Value=ZERO_INT
  Constant22 : Constant  Value=ENUM_PWRSTASW_OFF
  Constant{23,42,52,54} (4 alike) : Constant  Value=TRUE
  Constant24 : Constant  Value=KDDM_FRDoorSWPassTO_s
  Constant25 : Constant  Value=KDDM_FRDoorSWDTC_cnt
  Constant26 : Constant  Value=ONE_INT
  Constant32 : Constant  Value=ZERO_FLOAT
  Constant45 : Constant  Value=ENUM_POWERSTA_OFF
  Constant56 : Constant  Value=KDDM_FRDoorSWPassSW_flg
  Constant57 : Constant  Value=KDDM_FRDoorSWCFSSW_flg
  Constant58 : Constant  Value=KDDM_FRDoorSWDFSSW_flg
  Constant59 : Constant  Value=KDDM_FRDoorSWDetSW_flg
  Constant60 : Constant  Value=KDDM_FRDoorSWDTC_cnt
  DTC_Couter1 : hcu_lib/Basic_Blocks/DTC_Couter
  DTC_Info : hcu_lib/Basic_Blocks/DTC_Info
  Data Type Conversion12 : DataTypeConversion  OutDataTypeStr=boolean
  Data Type Conversion14 : DataTypeConversion  OutDataTypeStr=boolean
  Data Type Conversion4 : DataTypeConversion  OutDataTypeStr=uint8
  Data Type Conversion7 : DataTypeConversion
  Equal1 : RelationalOperator  Operator=~=  OutDataTypeStr=boolean  RndMeth=Simplest
  Equal3 : RelationalOperator  Operator=~=  OutDataTypeStr=boolean  RndMeth=Simplest
  Equal4 : RelationalOperator  Operator=~=  OutDataTypeStr=boolean  RndMeth=Simplest
  Equal5 : RelationalOperator  OutDataTypeStr=boolean  RndMeth=Simplest
  Equal8 : RelationalOperator  Operator===  OutDataTypeStr=boolean  RndMeth=Simplest
  Logical Operator{2,4..5,7} (4 alike) : Logic  Operator=NOT  AllPortsSameDT=off  OutDataTypeStr=boolean
  Logical Operator27 : Logic  Operator=OR  AllPortsSameDT=off  OutDataTypeStr=boolean
  Logical Operator{6,28..30} (4 alike) : Logic  AllPortsSameDT=off  OutDataTypeStr=boolean
  Logical Operator3 : Logic  Operator=OR  AllPortsSameDT=off  OutDataTypeStr=boolean
  Logical Operator31 : Logic  Inputs=3  AllPortsSameDT=off  OutDataTypeStr=boolean
  Logical Operator32 : Logic  Operator=OR  Inputs=3  AllPortsSameDT=off  OutDataTypeStr=boolean
  Logical Operator33 : Logic  Operator=OR  Inputs=3  AllPortsSameDT=off  OutDataTypeStr=boolean
  Relational Operator4 : RelationalOperator  Operator=<=  OutDataTypeStr=boolean  RndMeth=Simplest
  Relational Operator5 : RelationalOperator  Operator=>  OutDataTypeStr=boolean  RndMeth=Simplest
  Relay1 : Relay  OnSwitchValue=ONE_INT  OffSwitchValue=ZERO_INT
  SR_Latch1 : hcu_lib/Basic_Blocks/SR_Latch
  SR_Latch2 : hcu_lib/Basic_Blocks/SR_Latch
  SR_Latch3 : $bdroot/DDM/DDM/PMM/SW failure/Driver seat switch failure/SR_Latch3
  SR_Latch5 : hcu_lib/Basic_Blocks/SR_Latch
  Subsystem : $bdroot/DDM/DDM/PMM/SW failure/Driver seat switch failure/Subsystem  SystemSampleTime=-1  VariantActivationTime=update diagram  Latency=0  AutoFrameSizeCalculation=off
      link override Constant15: Value=KDDM_FRDoorSW_s
  Switch{5,10..11,14..16} (6 alike) : Switch  Criteria=u2 ~= 0
  Test Detection Criteria2 : hcu_lib/Basic_Blocks/Test Detection Criteria
  Timer : hcu_lib/Basic_Blocks/Test Detection Criteria/Timer
  Timer1 : hcu_lib/Basic_Blocks/Timer
  Unit Delay : UnitDelay  SampleTime=-1  HasFrameUpgradeWarning=on
  Unit Delay9 : UnitDelay  SampleTime=-1  HasFrameUpgradeWarning=on
  VDDM_FRDoorSWDTC_raw32 : Outport
  VDDM_VCUFRDoorSta_flg : Outport  Port=2
  wires:
  DTC_Couter1/1 -> SR_Latch5/1
  [DTC_clear_request] -> Logical Operator33/3
  [DTC_clear_request] -> Logical Operator3/2
  Logical Operator2/1 -> Logical Operator31/3
  DTC_Couter1/2 -> Data Type Conversion4/1
  [DTC_clear_request] -> Logical Operator2/1
  [DTC_clear_request] -> Logical Operator32/3
  [VDDM_FRDoorSWCFSRls_flg] -> Logical Operator33/2
  Constant60/1 -> DTC_Couter1/3
  Logical Operator30/1 -> [VDDM_FRDoorSWCFS_flg]  "VDDM_FRDoorSWCFS_flg"
  Logical Operator31/1 -> DTC_Couter1/1
  [VDDM_FRDoorSWCFS_flg] -> Logical Operator32/2
  SR_Latch2/1 -> Logical Operator28/2
  [VDDM_FRDoorSWCFSRls_flg] -> Logical Operator3/1
  Logical Operator33/1 -> Logical Operator29/1
  [VDDM_FRDoorSWDTC_cnt] -> Relay1/1
  Logical Operator32/1 -> SR_Latch2/2
  [VDDM_FRDoorSWPass_flg] -> Logical Operator33/1
  Logical Operator3/1 -> SR_Latch5/2
  [VDDM_FRDoorSWDet_flg] -> Logical Operator31/1
  Logical Operator28/1 -> [VDDM_FRDoorSWDFS_flg]
  Logical Operator29/1 -> DTC_Couter1/2
  Constant58/1 -> Logical Operator28/1
  Constant56/1 -> Logical Operator29/2
  SR_Latch5/1 -> Logical Operator30/1
  Data Type Conversion4/1 -> [VDDM_FRDoorSWDTC_cnt]  "VDDM_FRDoorSWDTC_cnt"
  Relay1/1 -> SR_Latch2/1
  Constant59/1 -> Logical Operator31/2
  [VDDM_FRDoorSWDFSRls_flg] -> Logical Operator32/1
  Constant57/1 -> Logical Operator30/2
  [DTC_clear_request] -> DTC_Info/4
  [VDDM_FRDoorSWDet_flg] -> DTC_Info/1
  [VDDM_FRDoorSWCFS_flg] -> DTC_Info/3
  [VDDM_FRDoorSWPass_flg] -> DTC_Info/2
  DTC_Info/1 -> VDDM_FRDoorSWDTC_raw32/1  "VDDM_FRDoorSWDTC_raw32"
  Constant10/1 -> Switch11/3
  VPMM_PwrStaSW_enum/1 -> [VPMM_PwrStaSW_enum]
  VPMM_PowerSta_enum/1 -> [VPMM_PowerSta_enum]
  [VDDM_VCUFRDoorSta_flg] -> VDDM_VCUFRDoorSta_flg/1
  [VPMM_PowerSta_enum] -> Equal8/1
  Constant54/1 -> Switch15/1
  [DTC_clear_request] -> Logical Operator27/2
  Switch16/1 -> [VDDM_FRDoorSWDFSRls_flg]
  Switch15/1 -> [VDDM_FRDoorSWCFSRls_flg]  "VDDM_FRDoorSWCFSRls_flg"
  Constant55/1 -> Switch15/3
  Constant45/1 -> Equal8/2
  Constant53/1 -> Switch16/3
  [VDDM_FRDoorSWPass_flg] -> Switch16/2
  Equal8/1 -> Logical Operator27/1
  Constant52/1 -> Switch16/1
  Logical Operator27/1 -> Switch15/2
  Switch11/1 -> [VDDM_VCUFRDoorSta_flg]  "VDDM_VCUFRDoorSta_flg"
  Constant42/1 -> Switch11/1
  [VDDM_FRDoorSWCFS_flg] -> Switch11/2
  task_time_s/1 -> [task_time_s]
  VINP_FRAJARSW/1 -> [VINP_FR_AJAR_SW]
  DTC_clear_request/1 -> [DTC_clear_request]
  Data Type Conversion14/1 -> Equal4/1
  Constant23/1 -> Switch10/3
  [task_time_s] -> Timer1/3
  Constant22/1 -> Equal1/2
  [task_time_s] -> Timer/3
  Constant21/1 -> Switch14/3
  Constant26/1 -> SR_Latch1/1
  [task_time_s] -> Test Detection Criteria2/2
  [FRDoorSWFault_flg] -> Switch10/1
  Logical Operator7/1 -> Timer1/1
  Timer1/1 -> Equal5/1
  Logical Operator4/1 -> Timer/2
  Data Type Conversion12/1 -> Test Detection Criteria2/1
  Data Type Conversion7/1 -> Test Detection Criteria2/4
  [VDDM_xxx_flg] -> SR_Latch3/2
  Unit Delay/1 -> Subsystem/1
  Constant25/1 -> Test Detection Criteria2/3
  Constant24/1 -> Equal5/2
  Subsystem/1 -> Logical Operator6/1
  Equal1/1 -> Switch14/2
  [DTC_clear_request] -> Switch5/2
  Constant16/1 -> Data Type Conversion7/1
  [VPMM_PwrStaSW_enum] -> Equal3/1
  Constant11/1 -> Timer/4
  Switch5/1 -> Data Type Conversion12/1
  Switch14/1 -> [VDDM_xxx_flg], Switch5/3
  SR_Latch1/1 -> Logical Operator5/1, Logical Operator4/1, Timer/1
  Relational Operator4/1 -> Logical Operator6/2
  Constant18/1 -> Switch5/1
  SR_Latch3/1 -> [VDDM_FRDoorSWPass_flg]  "VDDM_FRDoorSWPass_flg"
  Equal5/1 -> SR_Latch3/1
  Constant17/1 -> Relational Operator4/2
  Constant15/1 -> Timer1/4
  Equal3/1 -> Switch10/2
  Logical Operator6/1 -> [FRDoorSWFault_flg], Switch14/1
  [VPMM_PwrStaSW_enum] -> Equal1/1
  Logical Operator5/1 -> Subsystem/Trigger
  [VDDM_FRDoorSWChange_flg] -> SR_Latch1/2
  Relational Operator5/1 -> Unit Delay9/1, Equal4/2
  Unit Delay9/1 -> Data Type Conversion14/1
  Timer/1 -> Relational Operator4/1, Unit Delay/1
  [VINP_FR_AJAR_SW] -> Relational Operator5/1
  Constant19/1 -> Equal3/2
  Equal4/1 -> [VDDM_FRDoorSWChange_flg]
  Switch10/1 -> Logical Operator7/1, Timer1/2
  Constant32/1 -> Relational Operator5/2
  Test Detection Criteria2/1 -> [VDDM_FRDoorSWDet_flg]  "VDDM_FRDoorSWDet_flg"
